simulink model "lab03"  (Simulink 10.3)
settings: Solver=FixedStepAuto  StartTime=0.0  StopTime=2  FixedStep=0.001768  RelTol=1e-3
values from neighbouring files (symbols this model uses):
  k_d_1 = 0.00257391045559    [lab03.mat]    (also in lab04.mat; lab05.mat; lab06.mat; lab07.mat)
  k_d_2 = 0.013301286878    [lab03.mat]    (also in lab04.mat; lab05.mat; lab06.mat; lab07.mat)
  k_d_3 = 0.0267105074061    [lab03.mat]    (also in lab04.mat; lab05.mat; lab06.mat; lab07.mat)
  k_p = 2    [lab02.mat]    (also in lab03.mat = 0.256097247605; lab04.mat = 0.137612608424; lab05.mat = 0.280842058008; lab06.mat = 0.012)
undefined symbols (not defined in the file or in its folder): G_p
settings Model: Creator=kisdev  LastModifiedBy=kisdev
settings SolverCC: AlgebraicLoopSolver=Auto
settings DataIOCC: SaveFormat=Dataset  SignalLoggingSaveFormat=Dataset  ReturnWorkspaceOutputs=on
settings OptimizationCC: ExpressionDepthLimit=128  LifeSpan=auto
settings DebuggingCC: UnderspecifiedInitializationDetection=Simplified  MergeDetectMultiDrivingBlocksExec=error  FcnCallInpInsideContextMsg=error  StateNameClashWarn=none  SFUnexpectedBacktrackingDiag=error  SFNoUnconditionalDefaultTransitionDiag=error  SFExecutionAtInitializationDiag=warning  SFMachineParentedDataDiag=error  ArithmeticOperatorsInVariantConditions=error
settings HardwareCC: ProdBitPerPointer=64  ProdBitPerSizeT=64  ProdBitPerPtrDiffT=64  ProdLargestAtomicFloat=Float  ProdIntDivRoundTo=Zero  ProdEndianess=LittleEndian  ProdWordSize=64  ProdHWDeviceType=Intel->x86-64 (Windows64)
settings ModelReferenceCC: PropagateSignalLabelsOutOfModel=on
settings SFSimCC: SimUseLocalCustomCode=on  CustomCodeUndefinedFunction=FilterOut
settings RTWCC: RTWUseLocalCustomCode=on
settings CodeAppCC: StateflowObjectComments=off
settings GRTTargetCC: TargetLangStandard=C99 (ISO)  CombineOutputUpdateFcns=on  GRTInterface=off
settings ConfigComp: CovMetricSettings=dwe  CovSaveCumulativeToWorkspaceVar=off  CovSaveSingleToWorkspaceVar=off  CovExternalEMLEnable=on

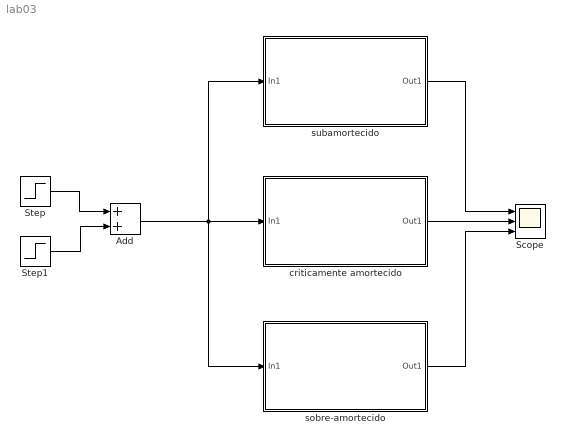
== system lab03 ==
  Add : Sum
  Scope : Scope  NumInputPorts=3
  Step : Step  Time=0  After=1000  SampleTime=0
  Step1 : Step  After=-2000  SampleTime=0
  criticamente amortecido : Subsystem
  sobre-amortecido : Subsystem
  subamortecido : Subsystem
  wires:
  Add/1 -> subamortecido/1(In1), sobre-amortecido/1(In1), criticamente amortecido/1(In1)
  criticamente amortecido/1(Out1) -> Scope/2
  sobre-amortecido/1(Out1) -> Scope/3
  Step/1 -> Add/1
  Step1/1 -> Add/2
  subamortecido/1(Out1) -> Scope/1

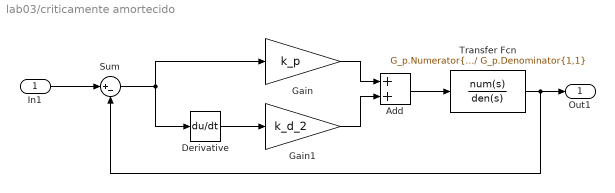
== system lab03/criticamente amortecido ==
  In1 : Inport
  Add : Sum
  Derivative : Derivative
  Gain : Gain  Gain=k_p
  Gain1 : Gain  Gain=k_d_2
  Sum : Sum  Inputs=|+-
  Transfer Fcn : TransferFcn  Numerator=G_p.Numerator{1,1}  Denominator=G_p.Denominator{1,1}
  Out1 : Outport
  wires:
  Transfer Fcn/1 -> Sum/2, Out1/1
  Gain/1 -> Add/1
  Gain1/1 -> Add/2
  Derivative/1 -> Gain1/1
  In1/1 -> Sum/1
  Sum/1 -> Derivative/1, Gain/1
  Add/1 -> Transfer Fcn/1

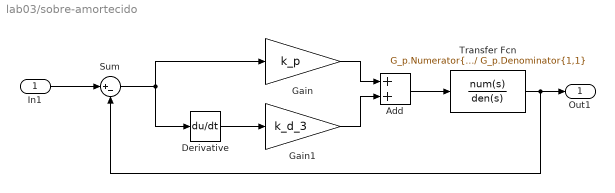
== system lab03/sobre-amortecido ==
  In1 : Inport
  Add : Sum
  Derivative : Derivative
  Gain : Gain  Gain=k_p
  Gain1 : Gain  Gain=k_d_3
  Sum : Sum  Inputs=|+-
  Transfer Fcn : TransferFcn  Numerator=G_p.Numerator{1,1}  Denominator=G_p.Denominator{1,1}
  Out1 : Outport
  wires:
  Transfer Fcn/1 -> Sum/2, Out1/1
  Gain/1 -> Add/1
  Gain1/1 -> Add/2
  Derivative/1 -> Gain1/1
  In1/1 -> Sum/1
  Sum/1 -> Derivative/1, Gain/1
  Add/1 -> Transfer Fcn/1

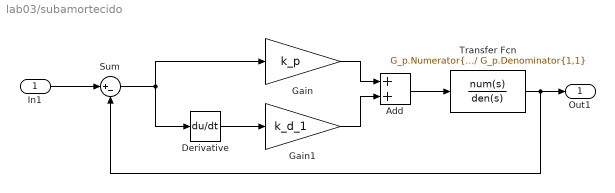
== system lab03/subamortecido ==
  In1 : Inport
  Add : Sum
  Derivative : Derivative
  Gain : Gain  Gain=k_p
  Gain1 : Gain  Gain=k_d_1
  Sum : Sum  Inputs=|+-
  Transfer Fcn : TransferFcn  Numerator=G_p.Numerator{1,1}  Denominator=G_p.Denominator{1,1}
  Out1 : Outport
  wires:
  Transfer Fcn/1 -> Sum/2, Out1/1
  Gain/1 -> Add/1
  Gain1/1 -> Add/2
  Derivative/1 -> Gain1/1
  In1/1 -> Sum/1
  Sum/1 -> Derivative/1, Gain/1
  Add/1 -> Transfer Fcn/1
